simulink model "Sixdof_model"  (R2024b)
settings: Solver=VariableStepAuto  StartTime=0.0  StopTime=50  RelTol=1e-3
values from neighbouring files (symbols this model uses):
  K_att = K_aug(:, 1:6)    [linear_model.m]
  K_I = K_aug(:, 7)    [linear_model.m]
libraries: simulink_extras x4, shared6dof x1, aerolibanim x1
settings Model: Creator=akewi  LastModifiedBy=akewi

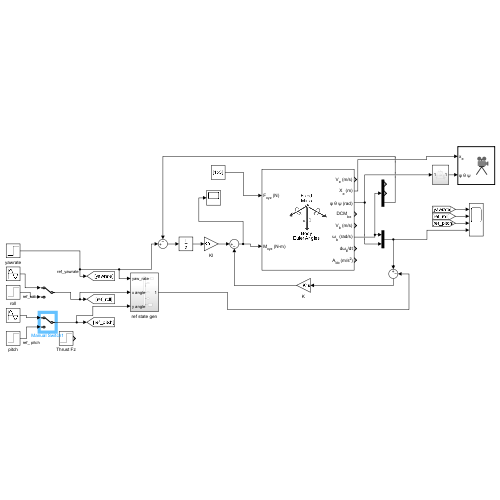
[thumbnail: Simulink's stored preview of the top-level diagram]
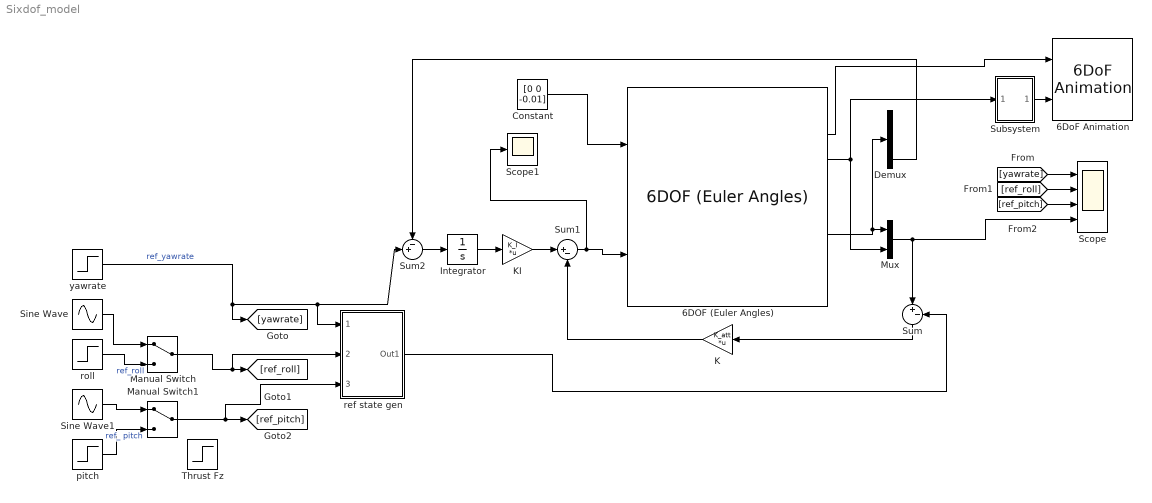
== system Sixdof_model ==
  6DOF (Euler Angles) : shared6dof/6DOF (Euler Angles)  units=Metric (MKS)  mtype=Fixed  rep=Euler Angles  xme_0=[0 0 0]  Vm_0=[0 0 0]  eul_0=[0 0 0]  pm_0=[0 0 0]  mass_0=1.0  mass_e=0.5  mass_f=2.0  inertia=Imatrix  inertia_e=eye(3)  inertia_f=2*eye(3)  k_quat=1.0  vre_flag=on  abi_flag=off  aMode=0  xme_statename=''  Vm_statename=''  eul_statename=''  quat_statename=''  pm_statename=''  mass_statename=''
  6DoF Animation : aerolibanim/6DoF Animation  u1=[-10 10 -10 10 -10 10]  u2=0.1  u3=5  u4=[10 10 0.1]  u5=Fixed position  u6=[2 2 1]  u7=110  u8=on
  Constant : Constant  Value=[0 0 -0.01]
  Demux : Demux  Outputs=3
  Integrator : Integrator
  K : Gain  Gain=K_att  Multiplication=Matrix(K*u)
  KI : Gain  Gain=K_I  Multiplication=Matrix(K*u)
  Manual Switch : ManualSwitch
  Manual Switch1 : ManualSwitch
  Mux : Mux  Inputs=2
  Scope : Scope  NumInputPorts=4
  Scope1 : Scope
  Sine Wave : Sin  Amplitude=45*pi/180  SampleTime=0
  Sine Wave1 : Sin  Amplitude=10*pi/180  Phase=pi  SampleTime=0
  Subsystem : Subsystem
  Sum : Sum  Inputs=|+-
  Sum1 : Sum  Inputs=|+-
  Sum2 : Sum  Inputs=-+|
  Thrust Fz : Step  SampleTime=0
  pitch : Step  After=10*pi/180  SampleTime=0
  ref state gen : Subsystem
  roll : Step  Time=3  After=10*pi/180  SampleTime=0
  yawrate : Step  Time=5  After=25*pi/180  SampleTime=0
  wires:
  yawrate/1 -> [yawrate], ref state gen/1(yaw_rate), Sum2/2  "ref_yawrate"
  [ref_roll] -> Scope/2
  [ref_pitch] -> Scope/3
  Mux/1 -> Sum/1, Scope/4
  [yawrate] -> Scope/1
  6DOF (Euler Angles)/6 -> Demux/1, Mux/1
  6DOF (Euler Angles)/3 -> Subsystem/1(In1), Mux/2
  Sum2/1 -> Integrator/1
  K/1 -> Sum1/2
  Integrator/1 -> KI/1
  Sum1/1 -> Scope1/1, 6DOF (Euler Angles)/2
  Sum/1 -> K/1
  ref state gen/1(Out1) -> Sum/2
  Demux/3 -> Sum2/1
  KI/1 -> Sum1/1
  6DOF (Euler Angles)/2 -> 6DoF Animation/1
  Subsystem/1(Out1) -> 6DoF Animation/2
  Manual Switch/1 -> ref state gen/2(x angle), [ref_roll]
  roll/1 -> Manual Switch/2  "ref_roll"
  Sine Wave/1 -> Manual Switch/1
  Manual Switch1/1 -> ref state gen/3(y angle), [ref_pitch]
  Sine Wave1/1 -> Manual Switch1/1
  pitch/1 -> Manual Switch1/2  "ref_ pitch"
  Constant/1 -> 6DOF (Euler Angles)/1

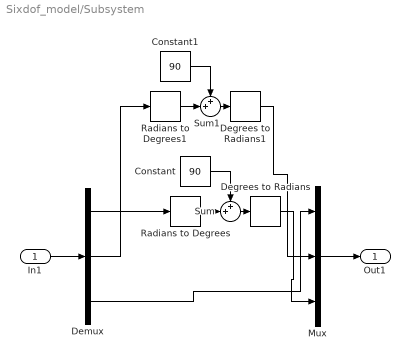
== system Sixdof_model/Subsystem ==
  In1 : Inport
  Constant : Constant  Value=90
  Constant1 : Constant  Value=90
  Degrees to Radians : simulink_extras/Transformations/Degrees to Radians
  Degrees to Radians1 : simulink_extras/Transformations/Degrees to Radians
  Demux : Demux  Outputs=3
  Mux : Mux  Inputs=3
  Radians to Degrees : simulink_extras/Transformations/Radians to Degrees
  Radians to Degrees1 : simulink_extras/Transformations/Radians to Degrees
  Sum : Sum  Inputs=++|
  Sum1 : Sum  Inputs=++|
  Out1 : Outport
  wires:
  Demux/1 -> Radians to Degrees/1
  Radians to Degrees/1 -> Sum/2
  Constant/1 -> Sum/1
  Sum/1 -> Degrees to Radians/1
  In1/1 -> Demux/1
  Mux/1 -> Out1/1
  Degrees to Radians/1 -> Mux/3
  Demux/3 -> Mux/1
  Degrees to Radians1/1 -> Mux/2
  Sum1/1 -> Degrees to Radians1/1
  Demux/2 -> Radians to Degrees1/1
  Radians to Degrees1/1 -> Sum1/2
  Constant1/1 -> Sum1/1

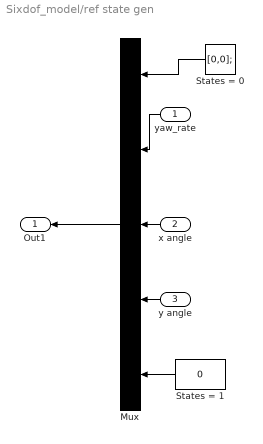
== system Sixdof_model/ref state gen ==
  yaw_rate : Inport
  x angle : Inport  Port=2
  y angle : Inport  Port=3
  Mux : Mux  Inputs=5
  States = 0 : Constant  Value=[0,0];
  States = 1 : Constant  Value=0
  Out1 : Outport
  wires:
  x angle/1 -> Mux/3
  States = 1/1 -> Mux/5
  y angle/1 -> Mux/4
  States = 0/1 -> Mux/1
  yaw_rate/1 -> Mux/2
  Mux/1 -> Out1/1
